simulink model "SendFetchS"  (Simulink 7.1)
settings: Solver=FixedStepDiscrete  StartTime=0.0  StopTime=5.0  FixedStep=0.1  RelTol=1e-3
libraries: simulink x1
settings Model: Creator=kthwsnt  LastModifiedBy=kthwsnt

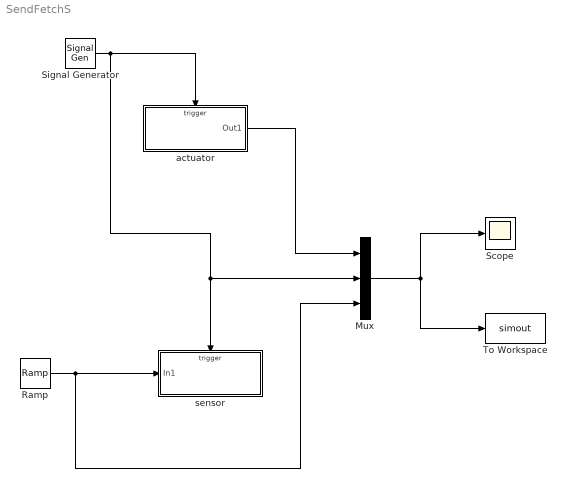
== system SendFetchS ==
  Mux : Mux  Inputs=3
  Ramp : simulink/Sources/Ramp  SystemSampleTime=-1  slope=2  start=0  X0=1
  Scope : Scope
      settings: TimeRange=10  YMax=10
  Signal Generator : SignalGenerator  WaveForm=square
  To Workspace : ToWorkspace  VariableName=simout  SampleTime=-1  SaveFormat=Structure
  actuator : Subsystem  TreatAsAtomicUnit=on
  sensor : Subsystem  TreatAsAtomicUnit=on
  wires:
  Signal Generator/1 -> Mux/2, sensor/Trigger, actuator/Trigger
  Mux/1 -> Scope/1, To Workspace/1
  actuator/1(Out1) -> Mux/1
  Ramp/1 -> sensor/1(In1), Mux/3

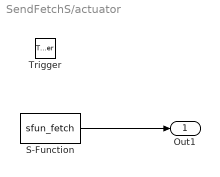
== system SendFetchS/actuator ==
  Trigger : TriggerPort  TriggerType=falling
  S-Function : S-Function  FunctionName=sfun_fetch  SFunctionModules='sfsource'  EnableBusSupport=off
  Out1 : Outport  OutDataType=sfix(16)  OutScaling=2^0
  wires:
  S-Function/1 -> Out1/1

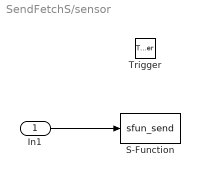
== system SendFetchS/sensor ==
  In1 : Inport  OutDataType=sfix(16)  OutScaling=2^0
  Trigger : TriggerPort
  S-Function : S-Function  FunctionName=sfun_send  SFunctionModules='sfsource'  EnableBusSupport=off
  wires:
  In1/1 -> S-Function/1
